simulink model "z_1.25"  (R2022b)
settings: Solver=VariableStepAuto  StartTime=0.0  StopTime=10.0  RelTol=1e-3
libraries: simulink x3
settings Model: Creator=amirz  LastModifiedBy=amirz

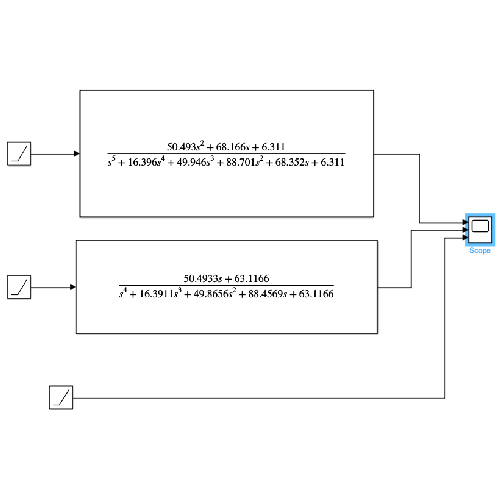
[thumbnail: Simulink's stored preview of the top-level diagram]
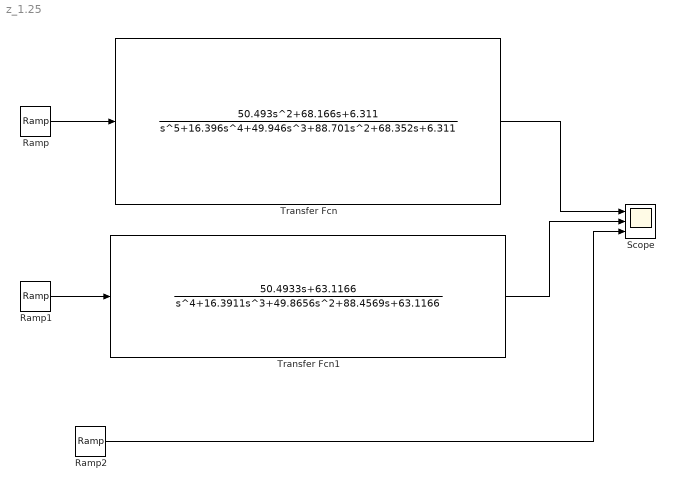
== system z_1.25 ==
  Ramp : simulink/Sources/Ramp  slope=1  start=0  InitialOutput=0
  Ramp1 : simulink/Sources/Ramp  slope=1  start=0  InitialOutput=0
  Ramp2 : simulink/Sources/Ramp  slope=1  start=0  InitialOutput=0
  Scope : Scope  NumInputPorts=3
  Transfer Fcn : TransferFcn  Numerator=[50.493 68.166 6.311]  Denominator=[1 16.396 49.946 88.701 68.352 6.311]
  Transfer Fcn1 : TransferFcn  Numerator=[50.4933 63.1166]  Denominator=[1 16.3911 49.8656 88.4569 63.1166]
  wires:
  Ramp/1 -> Transfer Fcn/1
  Ramp1/1 -> Transfer Fcn1/1
  Transfer Fcn/1 -> Scope/1
  Transfer Fcn1/1 -> Scope/2
  Ramp2/1 -> Scope/3
